simulink model "adrc_validation"  (R2026a)
settings: Solver=FixedStepDiscrete  StartTime=0  StopTime=6  FixedStep=0.004
model workspace (MAT data in the model file):
  scenarioB0 = 10
  scenarioDamping = 1
  scenarioDelay = 0
libraries: simulink x1
settings Model: Creator=Aethor_ca  LastModifiedBy=Aethor_ca
settings DebuggingCC: AlgebraicLoopMsg=error

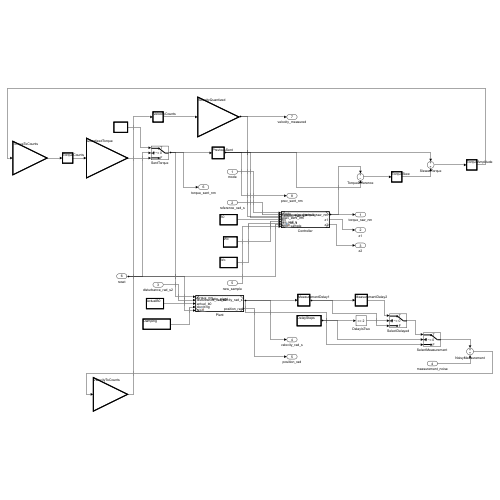
[thumbnail: Simulink's stored preview of the top-level diagram]
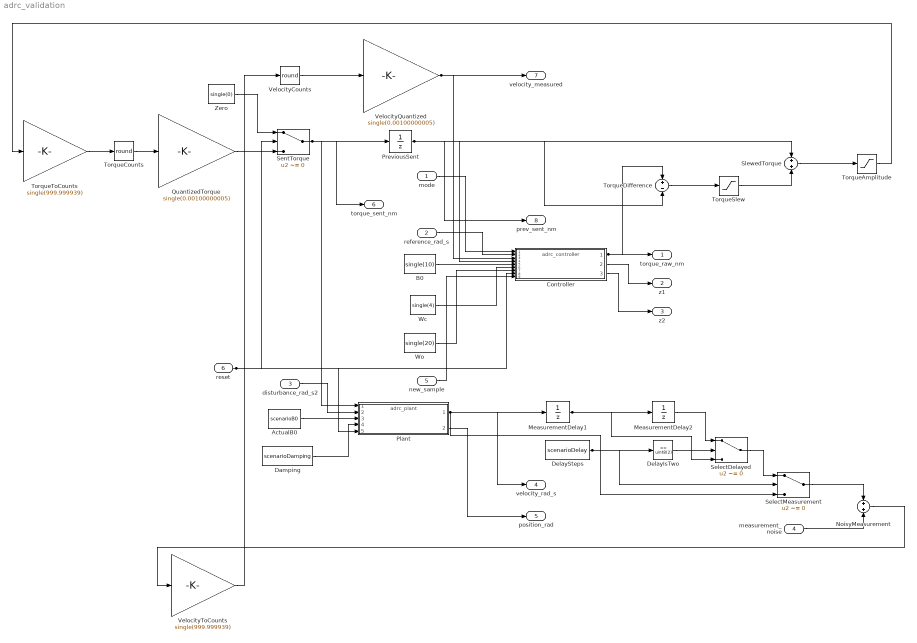
== system adrc_validation ==
  mode : Inport  OutDataTypeStr=uint8  PortDimensions=1  SampleTime=0.004
  reference_rad_s : Inport  Port=2  OutDataTypeStr=single  PortDimensions=1  SampleTime=0.004
  disturbance_rad_s2 : Inport  Port=3  OutDataTypeStr=single  PortDimensions=1  SampleTime=0.004
  measurement_noise : Inport  Port=4  OutDataTypeStr=single  PortDimensions=1  SampleTime=0.004
  new_sample : Inport  Port=5  OutDataTypeStr=uint8  PortDimensions=1  SampleTime=0.004
  reset : Inport  Port=6  OutDataTypeStr=uint8  PortDimensions=1  SampleTime=0.004
  ActualB0 : Constant  Value=scenarioB0  OutDataTypeStr=single
  B0 : Constant  Value=single(10)  OutDataTypeStr=single
  Controller : ModelReference  ModelNameDialog=adrc_controller  SimulationMode=Normal  ModelReferenceVersion=1.2
  Damping : Constant  Value=scenarioDamping  OutDataTypeStr=single
  DelayIsTwo : simulink/Logic and Bit Operations/Compare To Constant  relop===  const=uint8(2)  OutDataTypeStr=boolean
  DelaySteps : Constant  Value=scenarioDelay  OutDataTypeStr=uint8
  MeasurementDelay1 : UnitDelay  InitialCondition=single(0)  SampleTime=0.004
  MeasurementDelay2 : UnitDelay  InitialCondition=single(0)  SampleTime=0.004
  NoisyMeasurement : Sum  OutDataTypeStr=single
  Plant : ModelReference  ModelNameDialog=adrc_plant  SimulationMode=Normal  ModelReferenceVersion=1.2
  PreviousSent : UnitDelay  InitialCondition=single(0)  SampleTime=0.004
  QuantizedTorque : Gain  Gain=single(0.00100000005)  OutDataTypeStr=single
  SelectDelayed : Switch  Criteria=u2 ~= 0  OutDataTypeStr=single  SaturateOnIntegerOverflow=off  InputSameDT=off
  SelectMeasurement : Switch  Criteria=u2 ~= 0  OutDataTypeStr=single  SaturateOnIntegerOverflow=off  InputSameDT=off
  SentTorque : Switch  Criteria=u2 ~= 0  OutDataTypeStr=single  SaturateOnIntegerOverflow=off  InputSameDT=off
  SlewedTorque : Sum  OutDataTypeStr=single
  TorqueAmplitude : Saturate  UpperLimit=single(0.100000001)  LowerLimit=single(-0.100000001)
  TorqueCounts : Rounding  Operator=round
  TorqueDifference : Sum  Inputs=+-  OutDataTypeStr=single
  TorqueSlew : Saturate  UpperLimit=single(0.00200000009)  LowerLimit=single(-0.00200000009)
  TorqueToCounts : Gain  Gain=single(999.999939)  OutDataTypeStr=single
  VelocityCounts : Rounding  Operator=round
  VelocityQuantized : Gain  Gain=single(0.00100000005)  OutDataTypeStr=single
  VelocityToCounts : Gain  Gain=single(999.999939)  OutDataTypeStr=single
  Wc : Constant  Value=single(4)  OutDataTypeStr=single
  Wo : Constant  Value=single(20)  OutDataTypeStr=single
  Zero : Constant  Value=single(0)  OutDataTypeStr=single
  torque_raw_nm : Outport  OutDataTypeStr=single
  z1 : Outport  Port=2  OutDataTypeStr=single
  z2 : Outport  Port=3  OutDataTypeStr=single
  velocity_rad_s : Outport  Port=4  OutDataTypeStr=single
  position_rad : Outport  Port=5  OutDataTypeStr=single
  torque_sent_nm : Outport  Port=6  OutDataTypeStr=single
  velocity_measured : Outport  Port=7  OutDataTypeStr=single
  prev_sent_nm : Outport  Port=8  OutDataTypeStr=single
  wires:
  QuantizedTorque/1 -> SentTorque/3
  TorqueToCounts/1 -> TorqueCounts/1
  Controller/1 -> torque_raw_nm/1, TorqueDifference/1
  TorqueCounts/1 -> QuantizedTorque/1
  NoisyMeasurement/1 -> VelocityToCounts/1
  Zero/1 -> SentTorque/1
  reset/1 -> Controller/8, Plant/5, SentTorque/2
  Plant/2 -> position_rad/1
  SentTorque/1 -> PreviousSent/1, Plant/1, torque_sent_nm/1
  VelocityToCounts/1 -> VelocityCounts/1
  VelocityCounts/1 -> VelocityQuantized/1
  Controller/2 -> z1/1
  disturbance_rad_s2/1 -> Plant/2
  ActualB0/1 -> Plant/3
  Damping/1 -> Plant/4
  VelocityQuantized/1 -> Controller/3, velocity_measured/1
  PreviousSent/1 -> TorqueDifference/2, SlewedTorque/1, Controller/4, prev_sent_nm/1
  mode/1 -> Controller/1
  reference_rad_s/1 -> Controller/2
  B0/1 -> Controller/5
  SelectDelayed/1 -> SelectMeasurement/1
  Wc/1 -> Controller/6
  Wo/1 -> Controller/7
  new_sample/1 -> Controller/9
  Plant/1 -> SelectMeasurement/3, velocity_rad_s/1, MeasurementDelay1/1
  Controller/3 -> z2/1
  MeasurementDelay1/1 -> MeasurementDelay2/1, SelectDelayed/3
  DelaySteps/1 -> SelectMeasurement/2, DelayIsTwo/1
  TorqueDifference/1 -> TorqueSlew/1
  SlewedTorque/1 -> TorqueAmplitude/1
  MeasurementDelay2/1 -> SelectDelayed/1
  DelayIsTwo/1 -> SelectDelayed/2
  TorqueSlew/1 -> SlewedTorque/2
  SelectMeasurement/1 -> NoisyMeasurement/1
  measurement_noise/1 -> NoisyMeasurement/2
  TorqueAmplitude/1 -> TorqueToCounts/1
